simulink model "problem3"  (R2025b)
settings: Solver=VariableStepAuto  StartTime=0.0  StopTime=40.0  RelTol=1e-3
settings Model: Creator=Maria Islam  LastModifiedBy=Maria Islam

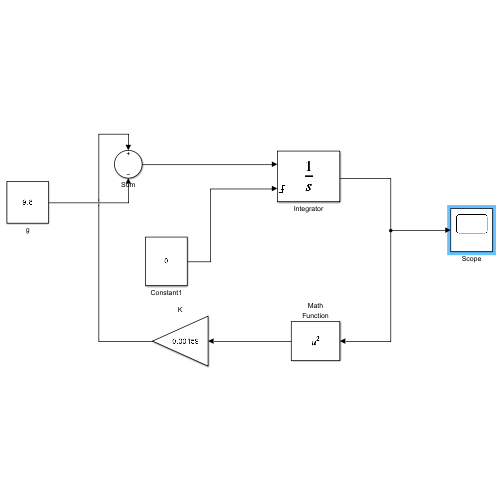
[thumbnail: Simulink's stored preview of the top-level diagram]
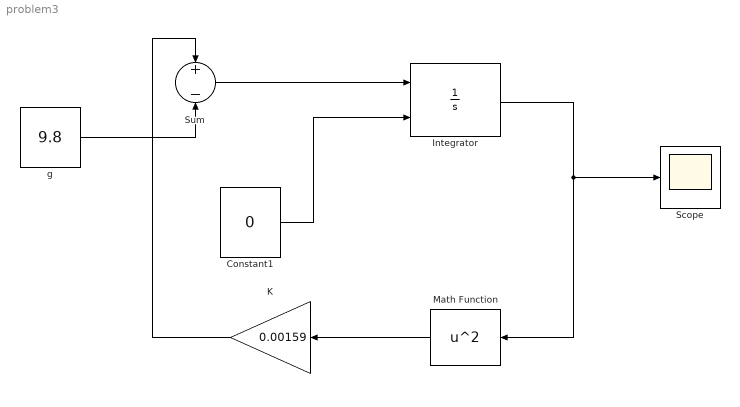
== system problem3 ==
  Constant1 : Constant  Value=0
  Integrator : Integrator  ExternalReset=rising
  K : Gain  Gain=0.00159
  Math Function : Math  Operator=square
  Scope : Scope
      settings: ActiveDisplayYMinimum=-88.313483857563  ActiveDisplayYMaximum=9.8126093175069986
  Sum : Sum  Inputs=+-
  g : Constant  Value=9.8
  wires:
  g/1 -> Sum/2
  Sum/1 -> Integrator/1
  K/1 -> Sum/1
  Constant1/1 -> Integrator/2
  Integrator/1 -> Math Function/1, Scope/1
  Math Function/1 -> K/1
